simulink library "sm_trackV_lib_belt_underc_elem"  (R2026a)
settings: Solver=VariableStepAuto
undefined symbols (not defined in the file): Excv, P00, P01, P02, P03, P04, P05, P06, P07, P08, P09, P10, P11, P12, P13, P14, P15, P16, P17, P18, P19, P20, Trac, X, Y, Z
libraries: sm_lib x193, $bdroot x42
(part 3 of 5)

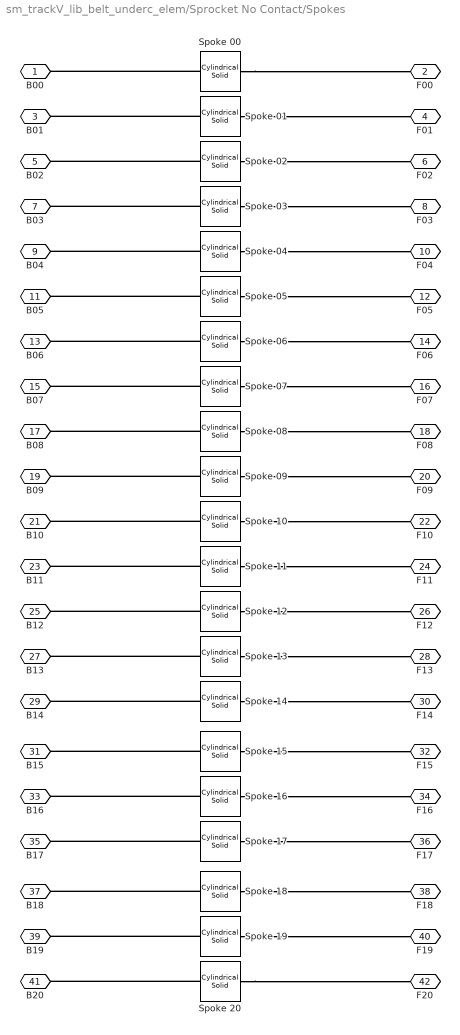
== system sm_trackV_lib_belt_underc_elem/Sprocket No Contact/Spokes ==
  Spoke 00 : sm_lib/Body Elements/Cylindrical Solid  CylinderRadius=sprk_spoke_rad  CylinderRadiusUnits=m  CylinderLength=sprk_spoke_len  CylinderLengthUnits=m  ExportEntireGeometry=off  InertiaType=PointMass  BasedOnType=Density  Density=1000  DensityUnits=kg/m^3  Mass=0  MassUnits=kg  CenterOfMass=[0 0 0]  CenterOfMassUnits=m  MomentsOfInertia=[1 1 1]  MomentsOfInertiaUnits=kg*m^2  ProductsOfInertia=[0 0 0]  ProductsOfInertiaUnits=kg*m^2  GraphicType=FromGeometry  MarkerShape=Sphere  MarkerSize=10  GraphicVisPropType=SimpleVisualProperties  GraphicDiffuseColor=sprk_spoke_clr  GraphicOpacity=sprk_spoke_opc  GraphicSpecularColor=[0.5 0.5 0.5 1.0]  GraphicAmbientColor=[0.15 0.15 0.15 1.0]  GraphicEmissiveColor=[0.0 0.0 0.0 1.0]  GraphicShininess=75  DoExposeReferenceFrame=on  SerializedFrames=<Frames><Frame><Id>Frame1</Id><Value><Name>C</Name><Origin><Source>GeometricFeature</Source><FeatureName>side surface</FeatureName></Origin><PrimaryAxis><DefinedDirection>+Z</DefinedDirection><Source>ReferenceFrame</Source><SourceDirection>+Z</SourceDirection><FeatureName></FeatureName></PrimaryAxis><SecondaryAxis><DefinedDirection>+X</DefinedDirection><Source>ReferenceFrame</Source><SourceDirection>+X</SourceDirection><FeatureName></FeatureName></SecondaryAxis></Value></Frame></Frames>
  Spoke 01 : sm_lib/Body Elements/Cylindrical Solid  CylinderRadius=sprk_spoke_rad  CylinderRadiusUnits=m  CylinderLength=sprk_spoke_len  CylinderLengthUnits=m  ExportEntireGeometry=off  InertiaType=PointMass  BasedOnType=Density  Density=1000  DensityUnits=kg/m^3  Mass=0  MassUnits=kg  CenterOfMass=[0 0 0]  CenterOfMassUnits=m  MomentsOfInertia=[1 1 1]  MomentsOfInertiaUnits=kg*m^2  ProductsOfInertia=[0 0 0]  ProductsOfInertiaUnits=kg*m^2  GraphicType=FromGeometry  MarkerShape=Sphere  MarkerSize=10  GraphicVisPropType=SimpleVisualProperties  GraphicDiffuseColor=sprk_spoke_clr  GraphicOpacity=sprk_spoke_opc  GraphicSpecularColor=[0.5 0.5 0.5 1.0]  GraphicAmbientColor=[0.15 0.15 0.15 1.0]  GraphicEmissiveColor=[0.0 0.0 0.0 1.0]  GraphicShininess=75  DoExposeReferenceFrame=on  SerializedFrames=<Frames><Frame><Id>Frame1</Id><Value><Name>C</Name><Origin><Source>GeometricFeature</Source><FeatureName>side surface</FeatureName></Origin><PrimaryAxis><DefinedDirection>+Z</DefinedDirection><Source>ReferenceFrame</Source><SourceDirection>+Z</SourceDirection><FeatureName></FeatureName></PrimaryAxis><SecondaryAxis><DefinedDirection>+X</DefinedDirection><Source>ReferenceFrame</Source><SourceDirection>+X</SourceDirection><FeatureName></FeatureName></SecondaryAxis></Value></Frame></Frames>
  Spoke 02 : sm_lib/Body Elements/Cylindrical Solid  CylinderRadius=sprk_spoke_rad  CylinderRadiusUnits=m  CylinderLength=sprk_spoke_len  CylinderLengthUnits=m  ExportEntireGeometry=off  InertiaType=PointMass  BasedOnType=Density  Density=1000  DensityUnits=kg/m^3  Mass=0  MassUnits=kg  CenterOfMass=[0 0 0]  CenterOfMassUnits=m  MomentsOfInertia=[1 1 1]  MomentsOfInertiaUnits=kg*m^2  ProductsOfInertia=[0 0 0]  ProductsOfInertiaUnits=kg*m^2  GraphicType=FromGeometry  MarkerShape=Sphere  MarkerSize=10  GraphicVisPropType=SimpleVisualProperties  GraphicDiffuseColor=sprk_spoke_clr  GraphicOpacity=sprk_spoke_opc  GraphicSpecularColor=[0.5 0.5 0.5 1.0]  GraphicAmbientColor=[0.15 0.15 0.15 1.0]  GraphicEmissiveColor=[0.0 0.0 0.0 1.0]  GraphicShininess=75  DoExposeReferenceFrame=on  SerializedFrames=<Frames><Frame><Id>Frame1</Id><Value><Name>C</Name><Origin><Source>GeometricFeature</Source><FeatureName>side surface</FeatureName></Origin><PrimaryAxis><DefinedDirection>+Z</DefinedDirection><Source>ReferenceFrame</Source><SourceDirection>+Z</SourceDirection><FeatureName></FeatureName></PrimaryAxis><SecondaryAxis><DefinedDirection>+X</DefinedDirection><Source>ReferenceFrame</Source><SourceDirection>+X</SourceDirection><FeatureName></FeatureName></SecondaryAxis></Value></Frame></Frames>
  Spoke 03 : sm_lib/Body Elements/Cylindrical Solid  CylinderRadius=sprk_spoke_rad  CylinderRadiusUnits=m  CylinderLength=sprk_spoke_len  CylinderLengthUnits=m  ExportEntireGeometry=off  InertiaType=PointMass  BasedOnType=Density  Density=1000  DensityUnits=kg/m^3  Mass=0  MassUnits=kg  CenterOfMass=[0 0 0]  CenterOfMassUnits=m  MomentsOfInertia=[1 1 1]  MomentsOfInertiaUnits=kg*m^2  ProductsOfInertia=[0 0 0]  ProductsOfInertiaUnits=kg*m^2  GraphicType=FromGeometry  MarkerShape=Sphere  MarkerSize=10  GraphicVisPropType=SimpleVisualProperties  GraphicDiffuseColor=sprk_spoke_clr  GraphicOpacity=sprk_spoke_opc  GraphicSpecularColor=[0.5 0.5 0.5 1.0]  GraphicAmbientColor=[0.15 0.15 0.15 1.0]  GraphicEmissiveColor=[0.0 0.0 0.0 1.0]  GraphicShininess=75  DoExposeReferenceFrame=on  SerializedFrames=<Frames><Frame><Id>Frame1</Id><Value><Name>C</Name><Origin><Source>GeometricFeature</Source><FeatureName>side surface</FeatureName></Origin><PrimaryAxis><DefinedDirection>+Z</DefinedDirection><Source>ReferenceFrame</Source><SourceDirection>+Z</SourceDirection><FeatureName></FeatureName></PrimaryAxis><SecondaryAxis><DefinedDirection>+X</DefinedDirection><Source>ReferenceFrame</Source><SourceDirection>+X</SourceDirection><FeatureName></FeatureName></SecondaryAxis></Value></Frame></Frames>
  Spoke 04 : sm_lib/Body Elements/Cylindrical Solid  CylinderRadius=sprk_spoke_rad  CylinderRadiusUnits=m  CylinderLength=sprk_spoke_len  CylinderLengthUnits=m  ExportEntireGeometry=off  InertiaType=PointMass  BasedOnType=Density  Density=1000  DensityUnits=kg/m^3  Mass=0  MassUnits=kg  CenterOfMass=[0 0 0]  CenterOfMassUnits=m  MomentsOfInertia=[1 1 1]  MomentsOfInertiaUnits=kg*m^2  ProductsOfInertia=[0 0 0]  ProductsOfInertiaUnits=kg*m^2  GraphicType=FromGeometry  MarkerShape=Sphere  MarkerSize=10  GraphicVisPropType=SimpleVisualProperties  GraphicDiffuseColor=sprk_spoke_clr  GraphicOpacity=sprk_spoke_opc  GraphicSpecularColor=[0.5 0.5 0.5 1.0]  GraphicAmbientColor=[0.15 0.15 0.15 1.0]  GraphicEmissiveColor=[0.0 0.0 0.0 1.0]  GraphicShininess=75  DoExposeReferenceFrame=on  SerializedFrames=<Frames><Frame><Id>Frame1</Id><Value><Name>C</Name><Origin><Source>GeometricFeature</Source><FeatureName>side surface</FeatureName></Origin><PrimaryAxis><DefinedDirection>+Z</DefinedDirection><Source>ReferenceFrame</Source><SourceDirection>+Z</SourceDirection><FeatureName></FeatureName></PrimaryAxis><SecondaryAxis><DefinedDirection>+X</DefinedDirection><Source>ReferenceFrame</Source><SourceDirection>+X</SourceDirection><FeatureName></FeatureName></SecondaryAxis></Value></Frame></Frames>
  Spoke 05 : sm_lib/Body Elements/Cylindrical Solid  CylinderRadius=sprk_spoke_rad  CylinderRadiusUnits=m  CylinderLength=sprk_spoke_len  CylinderLengthUnits=m  ExportEntireGeometry=off  InertiaType=PointMass  BasedOnType=Density  Density=1000  DensityUnits=kg/m^3  Mass=0  MassUnits=kg  CenterOfMass=[0 0 0]  CenterOfMassUnits=m  MomentsOfInertia=[1 1 1]  MomentsOfInertiaUnits=kg*m^2  ProductsOfInertia=[0 0 0]  ProductsOfInertiaUnits=kg*m^2  GraphicType=FromGeometry  MarkerShape=Sphere  MarkerSize=10  GraphicVisPropType=SimpleVisualProperties  GraphicDiffuseColor=sprk_spoke_clr  GraphicOpacity=sprk_spoke_opc  GraphicSpecularColor=[0.5 0.5 0.5 1.0]  GraphicAmbientColor=[0.15 0.15 0.15 1.0]  GraphicEmissiveColor=[0.0 0.0 0.0 1.0]  GraphicShininess=75  DoExposeReferenceFrame=on  SerializedFrames=<Frames><Frame><Id>Frame1</Id><Value><Name>C</Name><Origin><Source>GeometricFeature</Source><FeatureName>side surface</FeatureName></Origin><PrimaryAxis><DefinedDirection>+Z</DefinedDirection><Source>ReferenceFrame</Source><SourceDirection>+Z</SourceDirection><FeatureName></FeatureName></PrimaryAxis><SecondaryAxis><DefinedDirection>+X</DefinedDirection><Source>ReferenceFrame</Source><SourceDirection>+X</SourceDirection><FeatureName></FeatureName></SecondaryAxis></Value></Frame></Frames>
  Spoke 06 : sm_lib/Body Elements/Cylindrical Solid  CylinderRadius=sprk_spoke_rad  CylinderRadiusUnits=m  CylinderLength=sprk_spoke_len  CylinderLengthUnits=m  ExportEntireGeometry=off  InertiaType=PointMass  BasedOnType=Density  Density=1000  DensityUnits=kg/m^3  Mass=0  MassUnits=kg  CenterOfMass=[0 0 0]  CenterOfMassUnits=m  MomentsOfInertia=[1 1 1]  MomentsOfInertiaUnits=kg*m^2  ProductsOfInertia=[0 0 0]  ProductsOfInertiaUnits=kg*m^2  GraphicType=FromGeometry  MarkerShape=Sphere  MarkerSize=10  GraphicVisPropType=SimpleVisualProperties  GraphicDiffuseColor=sprk_spoke_clr  GraphicOpacity=sprk_spoke_opc  GraphicSpecularColor=[0.5 0.5 0.5 1.0]  GraphicAmbientColor=[0.15 0.15 0.15 1.0]  GraphicEmissiveColor=[0.0 0.0 0.0 1.0]  GraphicShininess=75  DoExposeReferenceFrame=on  SerializedFrames=<Frames><Frame><Id>Frame1</Id><Value><Name>C</Name><Origin><Source>GeometricFeature</Source><FeatureName>side surface</FeatureName></Origin><PrimaryAxis><DefinedDirection>+Z</DefinedDirection><Source>ReferenceFrame</Source><SourceDirection>+Z</SourceDirection><FeatureName></FeatureName></PrimaryAxis><SecondaryAxis><DefinedDirection>+X</DefinedDirection><Source>ReferenceFrame</Source><SourceDirection>+X</SourceDirection><FeatureName></FeatureName></SecondaryAxis></Value></Frame></Frames>
  Spoke 07 : sm_lib/Body Elements/Cylindrical Solid  CylinderRadius=sprk_spoke_rad  CylinderRadiusUnits=m  CylinderLength=sprk_spoke_len  CylinderLengthUnits=m  ExportEntireGeometry=off  InertiaType=PointMass  BasedOnType=Density  Density=1000  DensityUnits=kg/m^3  Mass=0  MassUnits=kg  CenterOfMass=[0 0 0]  CenterOfMassUnits=m  MomentsOfInertia=[1 1 1]  MomentsOfInertiaUnits=kg*m^2  ProductsOfInertia=[0 0 0]  ProductsOfInertiaUnits=kg*m^2  GraphicType=FromGeometry  MarkerShape=Sphere  MarkerSize=10  GraphicVisPropType=SimpleVisualProperties  GraphicDiffuseColor=sprk_spoke_clr  GraphicOpacity=sprk_spoke_opc  GraphicSpecularColor=[0.5 0.5 0.5 1.0]  GraphicAmbientColor=[0.15 0.15 0.15 1.0]  GraphicEmissiveColor=[0.0 0.0 0.0 1.0]  GraphicShininess=75  DoExposeReferenceFrame=on  SerializedFrames=<Frames><Frame><Id>Frame1</Id><Value><Name>C</Name><Origin><Source>GeometricFeature</Source><FeatureName>side surface</FeatureName></Origin><PrimaryAxis><DefinedDirection>+Z</DefinedDirection><Source>ReferenceFrame</Source><SourceDirection>+Z</SourceDirection><FeatureName></FeatureName></PrimaryAxis><SecondaryAxis><DefinedDirection>+X</DefinedDirection><Source>ReferenceFrame</Source><SourceDirection>+X</SourceDirection><FeatureName></FeatureName></SecondaryAxis></Value></Frame></Frames>
  Spoke 08 : sm_lib/Body Elements/Cylindrical Solid  CylinderRadius=sprk_spoke_rad  CylinderRadiusUnits=m  CylinderLength=sprk_spoke_len  CylinderLengthUnits=m  ExportEntireGeometry=off  InertiaType=PointMass  BasedOnType=Density  Density=1000  DensityUnits=kg/m^3  Mass=0  MassUnits=kg  CenterOfMass=[0 0 0]  CenterOfMassUnits=m  MomentsOfInertia=[1 1 1]  MomentsOfInertiaUnits=kg*m^2  ProductsOfInertia=[0 0 0]  ProductsOfInertiaUnits=kg*m^2  GraphicType=FromGeometry  MarkerShape=Sphere  MarkerSize=10  GraphicVisPropType=SimpleVisualProperties  GraphicDiffuseColor=sprk_spoke_clr  GraphicOpacity=sprk_spoke_opc  GraphicSpecularColor=[0.5 0.5 0.5 1.0]  GraphicAmbientColor=[0.15 0.15 0.15 1.0]  GraphicEmissiveColor=[0.0 0.0 0.0 1.0]  GraphicShininess=75  DoExposeReferenceFrame=on  SerializedFrames=<Frames><Frame><Id>Frame1</Id><Value><Name>C</Name><Origin><Source>GeometricFeature</Source><FeatureName>side surface</FeatureName></Origin><PrimaryAxis><DefinedDirection>+Z</DefinedDirection><Source>ReferenceFrame</Source><SourceDirection>+Z</SourceDirection><FeatureName></FeatureName></PrimaryAxis><SecondaryAxis><DefinedDirection>+X</DefinedDirection><Source>ReferenceFrame</Source><SourceDirection>+X</SourceDirection><FeatureName></FeatureName></SecondaryAxis></Value></Frame></Frames>
  Spoke 09 : sm_lib/Body Elements/Cylindrical Solid  CylinderRadius=sprk_spoke_rad  CylinderRadiusUnits=m  CylinderLength=sprk_spoke_len  CylinderLengthUnits=m  ExportEntireGeometry=off  InertiaType=PointMass  BasedOnType=Density  Density=1000  DensityUnits=kg/m^3  Mass=0  MassUnits=kg  CenterOfMass=[0 0 0]  CenterOfMassUnits=m  MomentsOfInertia=[1 1 1]  MomentsOfInertiaUnits=kg*m^2  ProductsOfInertia=[0 0 0]  ProductsOfInertiaUnits=kg*m^2  GraphicType=FromGeometry  MarkerShape=Sphere  MarkerSize=10  GraphicVisPropType=SimpleVisualProperties  GraphicDiffuseColor=sprk_spoke_clr  GraphicOpacity=sprk_spoke_opc  GraphicSpecularColor=[0.5 0.5 0.5 1.0]  GraphicAmbientColor=[0.15 0.15 0.15 1.0]  GraphicEmissiveColor=[0.0 0.0 0.0 1.0]  GraphicShininess=75  DoExposeReferenceFrame=on  SerializedFrames=<Frames><Frame><Id>Frame1</Id><Value><Name>C</Name><Origin><Source>GeometricFeature</Source><FeatureName>side surface</FeatureName></Origin><PrimaryAxis><DefinedDirection>+Z</DefinedDirection><Source>ReferenceFrame</Source><SourceDirection>+Z</SourceDirection><FeatureName></FeatureName></PrimaryAxis><SecondaryAxis><DefinedDirection>+X</DefinedDirection><Source>ReferenceFrame</Source><SourceDirection>+X</SourceDirection><FeatureName></FeatureName></SecondaryAxis></Value></Frame></Frames>
  Spoke {10..20} (11 alike) : sm_lib/Body Elements/Cylindrical Solid  CylinderRadius=sprk_spoke_rad  CylinderRadiusUnits=m  CylinderLength=sprk_spoke_len  CylinderLengthUnits=m  ExportEntireGeometry=off  InertiaType=PointMass  BasedOnType=Density  Density=1000  DensityUnits=kg/m^3  Mass=0  MassUnits=kg  CenterOfMass=[0 0 0]  CenterOfMassUnits=m  MomentsOfInertia=[1 1 1]  MomentsOfInertiaUnits=kg*m^2  ProductsOfInertia=[0 0 0]  ProductsOfInertiaUnits=kg*m^2  GraphicType=FromGeometry  MarkerShape=Sphere  MarkerSize=10  GraphicVisPropType=SimpleVisualProperties  GraphicDiffuseColor=sprk_spoke_clr  GraphicOpacity=sprk_spoke_opc  GraphicSpecularColor=[0.5 0.5 0.5 1.0]  GraphicAmbientColor=[0.15 0.15 0.15 1.0]  GraphicEmissiveColor=[0.0 0.0 0.0 1.0]  GraphicShininess=75  DoExposeReferenceFrame=on  SerializedFrames=<Frames><Frame><Id>Frame1</Id><Value><Name>C</Name><Origin><Source>GeometricFeature</Source><FeatureName>side surface</FeatureName></Origin><PrimaryAxis><DefinedDirection>+Z</DefinedDirection><Source>ReferenceFrame</Source><SourceDirection>+Z</SourceDirection><FeatureName></FeatureName></PrimaryAxis><SecondaryAxis><DefinedDirection>+X</DefinedDirection><Source>ReferenceFrame</Source><SourceDirection>+X</SourceDirection><FeatureName></FeatureName></SecondaryAxis></Value></Frame></Frames>
  B00 : PMIOPort  Side=Left
  F00 : PMIOPort  Port=2  Side=Right
  B01 : PMIOPort  Port=3  Side=Left
  F01 : PMIOPort  Port=4  Side=Right
  B02 : PMIOPort  Port=5  Side=Left
  F02 : PMIOPort  Port=6  Side=Right
  B03 : PMIOPort  Port=7  Side=Left
  F03 : PMIOPort  Port=8  Side=Right
  B04 : PMIOPort  Port=9  Side=Left
  F04 : PMIOPort  Port=10  Side=Right
  B05 : PMIOPort  Port=11  Side=Left
  F05 : PMIOPort  Port=12  Side=Right
  B06 : PMIOPort  Port=13  Side=Left
  F06 : PMIOPort  Port=14  Side=Right
  B07 : PMIOPort  Port=15  Side=Left
  F07 : PMIOPort  Port=16  Side=Right
  B08 : PMIOPort  Port=17  Side=Left
  F08 : PMIOPort  Port=18  Side=Right
  B09 : PMIOPort  Port=19  Side=Left
  F09 : PMIOPort  Port=20  Side=Right
  B10 : PMIOPort  Port=21  Side=Left
  F10 : PMIOPort  Port=22  Side=Right
  B11 : PMIOPort  Port=23  Side=Left
  F11 : PMIOPort  Port=24  Side=Right
  B12 : PMIOPort  Port=25  Side=Left
  F12 : PMIOPort  Port=26  Side=Right
  B13 : PMIOPort  Port=27  Side=Left
  F13 : PMIOPort  Port=28  Side=Right
  B14 : PMIOPort  Port=29  Side=Left
  F14 : PMIOPort  Port=30  Side=Right
  B15 : PMIOPort  Port=31  Side=Left
  F15 : PMIOPort  Port=32  Side=Right
  B16 : PMIOPort  Port=33  Side=Left
  F16 : PMIOPort  Port=34  Side=Right
  B17 : PMIOPort  Port=35  Side=Left
  F17 : PMIOPort  Port=36  Side=Right
  B18 : PMIOPort  Port=37  Side=Left
  F18 : PMIOPort  Port=38  Side=Right
  B19 : PMIOPort  Port=39  Side=Left
  F19 : PMIOPort  Port=40  Side=Right
  B20 : PMIOPort  Port=41  Side=Left
  F20 : PMIOPort  Port=42  Side=Right
  connections:
  Spoke 20/RConn1 -- F20/RConn1
  Spoke 08/RConn1 -- F08/RConn1
  Spoke 06/RConn1 -- F06/RConn1
  Spoke 02/RConn1 -- F02/RConn1
  Spoke 04/RConn1 -- F04/RConn1
  Spoke 14/RConn1 -- F14/RConn1
  Spoke 03/RConn1 -- F03/RConn1
  Spoke 17/RConn1 -- F17/RConn1
  Spoke 15/LConn1 -- B15/RConn1
  Spoke 20/LConn1 -- B20/RConn1
  Spoke 16/LConn1 -- B16/RConn1
  Spoke 04/LConn1 -- B04/RConn1
  Spoke 05/LConn1 -- B05/RConn1
  Spoke 14/LConn1 -- B14/RConn1
  Spoke 11/RConn1 -- F11/RConn1
  Spoke 11/LConn1 -- B11/RConn1
  Spoke 12/RConn1 -- F12/RConn1
  Spoke 18/RConn1 -- F18/RConn1
  Spoke 13/LConn1 -- B13/RConn1
  Spoke 02/LConn1 -- B02/RConn1
  Spoke 09/LConn1 -- B09/RConn1
  Spoke 19/LConn1 -- B19/RConn1
  Spoke 17/LConn1 -- B17/RConn1
  Spoke 18/LConn1 -- B18/RConn1
  Spoke 19/RConn1 -- F19/RConn1
  Spoke 05/RConn1 -- F05/RConn1
  Spoke 16/RConn1 -- F16/RConn1
  Spoke 09/RConn1 -- F09/RConn1
  Spoke 10/LConn1 -- B10/RConn1
  Spoke 07/LConn1 -- B07/RConn1
  Spoke 10/RConn1 -- F10/RConn1
  Spoke 07/RConn1 -- F07/RConn1
  Spoke 00/RConn1 -- F00/RConn1
  Spoke 01/LConn1 -- B01/RConn1
  Spoke 08/LConn1 -- B08/RConn1
  Spoke 12/LConn1 -- B12/RConn1
  Spoke 01/RConn1 -- F01/RConn1
  Spoke 15/RConn1 -- F15/RConn1
  Spoke 13/RConn1 -- F13/RConn1
  Spoke 06/LConn1 -- B06/RConn1
  Spoke 03/LConn1 -- B03/RConn1
  Spoke 00/LConn1 -- B00/RConn1

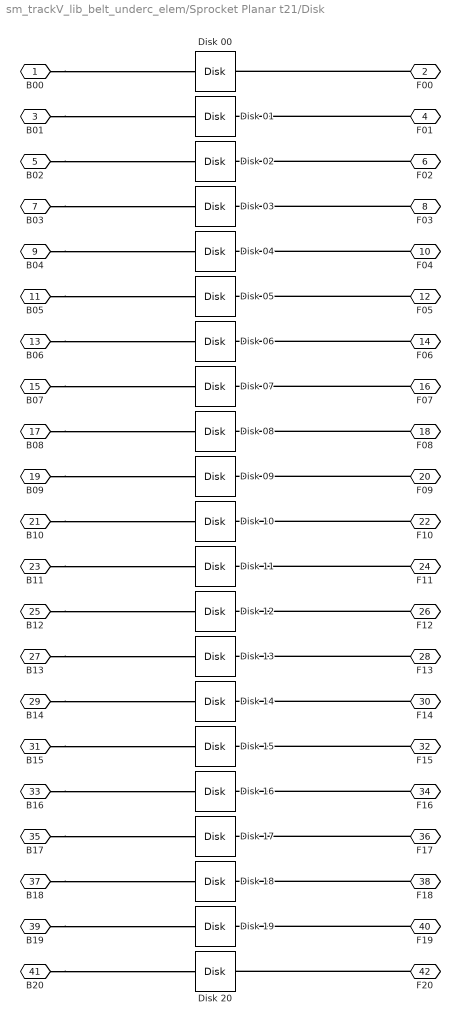
== system sm_trackV_lib_belt_underc_elem/Sprocket Planar t21/Disk ==
  Disk 00 : sm_lib/Curves and Surfaces/Disk  Radius=sprk_spoke_rad  RadiusUnits=m  GraphicType=FromGeometry  GraphicVisPropType=SimpleVisualProperties  GraphicDiffuseColor=sprk_contgeo_spoke_clr  GraphicOpacity=sprk_contgeo_spoke_opc  GraphicSpecularColor=[0.5 0.5 0.5 1.0]  GraphicAmbientColor=[0.15 0.15 0.15 1.0]  GraphicEmissiveColor=[0.0 0.0 0.0 1.0]  GraphicShininess=75
  Disk 01 : sm_lib/Curves and Surfaces/Disk  Radius=sprk_spoke_rad  RadiusUnits=m  GraphicType=FromGeometry  GraphicVisPropType=SimpleVisualProperties  GraphicDiffuseColor=sprk_contgeo_spoke_clr  GraphicOpacity=sprk_contgeo_spoke_opc  GraphicSpecularColor=[0.5 0.5 0.5 1.0]  GraphicAmbientColor=[0.15 0.15 0.15 1.0]  GraphicEmissiveColor=[0.0 0.0 0.0 1.0]  GraphicShininess=75
  Disk 02 : sm_lib/Curves and Surfaces/Disk  Radius=sprk_spoke_rad  RadiusUnits=m  GraphicType=FromGeometry  GraphicVisPropType=SimpleVisualProperties  GraphicDiffuseColor=sprk_contgeo_spoke_clr  GraphicOpacity=sprk_contgeo_spoke_opc  GraphicSpecularColor=[0.5 0.5 0.5 1.0]  GraphicAmbientColor=[0.15 0.15 0.15 1.0]  GraphicEmissiveColor=[0.0 0.0 0.0 1.0]  GraphicShininess=75
  Disk 03 : sm_lib/Curves and Surfaces/Disk  Radius=sprk_spoke_rad  RadiusUnits=m  GraphicType=FromGeometry  GraphicVisPropType=SimpleVisualProperties  GraphicDiffuseColor=sprk_contgeo_spoke_clr  GraphicOpacity=sprk_contgeo_spoke_opc  GraphicSpecularColor=[0.5 0.5 0.5 1.0]  GraphicAmbientColor=[0.15 0.15 0.15 1.0]  GraphicEmissiveColor=[0.0 0.0 0.0 1.0]  GraphicShininess=75
  Disk 04 : sm_lib/Curves and Surfaces/Disk  Radius=sprk_spoke_rad  RadiusUnits=m  GraphicType=FromGeometry  GraphicVisPropType=SimpleVisualProperties  GraphicDiffuseColor=sprk_contgeo_spoke_clr  GraphicOpacity=sprk_contgeo_spoke_opc  GraphicSpecularColor=[0.5 0.5 0.5 1.0]  GraphicAmbientColor=[0.15 0.15 0.15 1.0]  GraphicEmissiveColor=[0.0 0.0 0.0 1.0]  GraphicShininess=75
  Disk 05 : sm_lib/Curves and Surfaces/Disk  Radius=sprk_spoke_rad  RadiusUnits=m  GraphicType=FromGeometry  GraphicVisPropType=SimpleVisualProperties  GraphicDiffuseColor=sprk_contgeo_spoke_clr  GraphicOpacity=sprk_contgeo_spoke_opc  GraphicSpecularColor=[0.5 0.5 0.5 1.0]  GraphicAmbientColor=[0.15 0.15 0.15 1.0]  GraphicEmissiveColor=[0.0 0.0 0.0 1.0]  GraphicShininess=75
  Disk 06 : sm_lib/Curves and Surfaces/Disk  Radius=sprk_spoke_rad  RadiusUnits=m  GraphicType=FromGeometry  GraphicVisPropType=SimpleVisualProperties  GraphicDiffuseColor=sprk_contgeo_spoke_clr  GraphicOpacity=sprk_contgeo_spoke_opc  GraphicSpecularColor=[0.5 0.5 0.5 1.0]  GraphicAmbientColor=[0.15 0.15 0.15 1.0]  GraphicEmissiveColor=[0.0 0.0 0.0 1.0]  GraphicShininess=75
  Disk 07 : sm_lib/Curves and Surfaces/Disk  Radius=sprk_spoke_rad  RadiusUnits=m  GraphicType=FromGeometry  GraphicVisPropType=SimpleVisualProperties  GraphicDiffuseColor=sprk_contgeo_spoke_clr  GraphicOpacity=sprk_contgeo_spoke_opc  GraphicSpecularColor=[0.5 0.5 0.5 1.0]  GraphicAmbientColor=[0.15 0.15 0.15 1.0]  GraphicEmissiveColor=[0.0 0.0 0.0 1.0]  GraphicShininess=75
  Disk 08 : sm_lib/Curves and Surfaces/Disk  Radius=sprk_spoke_rad  RadiusUnits=m  GraphicType=FromGeometry  GraphicVisPropType=SimpleVisualProperties  GraphicDiffuseColor=sprk_contgeo_spoke_clr  GraphicOpacity=sprk_contgeo_spoke_opc  GraphicSpecularColor=[0.5 0.5 0.5 1.0]  GraphicAmbientColor=[0.15 0.15 0.15 1.0]  GraphicEmissiveColor=[0.0 0.0 0.0 1.0]  GraphicShininess=75
  Disk 09 : sm_lib/Curves and Surfaces/Disk  Radius=sprk_spoke_rad  RadiusUnits=m  GraphicType=FromGeometry  GraphicVisPropType=SimpleVisualProperties  GraphicDiffuseColor=sprk_contgeo_spoke_clr  GraphicOpacity=sprk_contgeo_spoke_opc  GraphicSpecularColor=[0.5 0.5 0.5 1.0]  GraphicAmbientColor=[0.15 0.15 0.15 1.0]  GraphicEmissiveColor=[0.0 0.0 0.0 1.0]  GraphicShininess=75
  Disk {10..20} (11 alike) : sm_lib/Curves and Surfaces/Disk  Radius=sprk_spoke_rad  RadiusUnits=m  GraphicType=FromGeometry  GraphicVisPropType=SimpleVisualProperties  GraphicDiffuseColor=sprk_contgeo_spoke_clr  GraphicOpacity=sprk_contgeo_spoke_opc  GraphicSpecularColor=[0.5 0.5 0.5 1.0]  GraphicAmbientColor=[0.15 0.15 0.15 1.0]  GraphicEmissiveColor=[0.0 0.0 0.0 1.0]  GraphicShininess=75
  B00 : PMIOPort  Side=Left
  F00 : PMIOPort  Port=2  Side=Right
  B01 : PMIOPort  Port=3  Side=Left
  F01 : PMIOPort  Port=4  Side=Right
  B02 : PMIOPort  Port=5  Side=Left
  F02 : PMIOPort  Port=6  Side=Right
  B03 : PMIOPort  Port=7  Side=Left
  F03 : PMIOPort  Port=8  Side=Right
  B04 : PMIOPort  Port=9  Side=Left
  F04 : PMIOPort  Port=10  Side=Right
  B05 : PMIOPort  Port=11  Side=Left
  F05 : PMIOPort  Port=12  Side=Right
  B06 : PMIOPort  Port=13  Side=Left
  F06 : PMIOPort  Port=14  Side=Right
  B07 : PMIOPort  Port=15  Side=Left
  F07 : PMIOPort  Port=16  Side=Right
  B08 : PMIOPort  Port=17  Side=Left
  F08 : PMIOPort  Port=18  Side=Right
  B09 : PMIOPort  Port=19  Side=Left
  F09 : PMIOPort  Port=20  Side=Right
  B10 : PMIOPort  Port=21  Side=Left
  F10 : PMIOPort  Port=22  Side=Right
  B11 : PMIOPort  Port=23  Side=Left
  F11 : PMIOPort  Port=24  Side=Right
  B12 : PMIOPort  Port=25  Side=Left
  F12 : PMIOPort  Port=26  Side=Right
  B13 : PMIOPort  Port=27  Side=Left
  F13 : PMIOPort  Port=28  Side=Right
  B14 : PMIOPort  Port=29  Side=Left
  F14 : PMIOPort  Port=30  Side=Right
  B15 : PMIOPort  Port=31  Side=Left
  F15 : PMIOPort  Port=32  Side=Right
  B16 : PMIOPort  Port=33  Side=Left
  F16 : PMIOPort  Port=34  Side=Right
  B17 : PMIOPort  Port=35  Side=Left
  F17 : PMIOPort  Port=36  Side=Right
  B18 : PMIOPort  Port=37  Side=Left
  F18 : PMIOPort  Port=38  Side=Right
  B19 : PMIOPort  Port=39  Side=Left
  F19 : PMIOPort  Port=40  Side=Right
  B20 : PMIOPort  Port=41  Side=Left
  F20 : PMIOPort  Port=42  Side=Right
  connections:
  B01/RConn1 -- Disk 01/LConn1
  F10/RConn1 -- Disk 10/RConn1
  B13/RConn1 -- Disk 13/LConn1
  B05/RConn1 -- Disk 05/LConn1
  B06/RConn1 -- Disk 06/LConn1
  B00/RConn1 -- Disk 00/LConn1
  F00/RConn1 -- Disk 00/RConn1
  B19/RConn1 -- Disk 19/LConn1
  B14/RConn1 -- Disk 14/LConn1
  B20/RConn1 -- Disk 20/LConn1
  B02/RConn1 -- Disk 02/LConn1
  B04/RConn1 -- Disk 04/LConn1
  B03/RConn1 -- Disk 03/LConn1
  B07/RConn1 -- Disk 07/LConn1
  F11/RConn1 -- Disk 11/RConn1
  B08/RConn1 -- Disk 08/LConn1
  F08/RConn1 -- Disk 08/RConn1
  B12/RConn1 -- Disk 12/LConn1
  B10/RConn1 -- Disk 10/LConn1
  B17/RConn1 -- Disk 17/LConn1
  B09/RConn1 -- Disk 09/LConn1
  B11/RConn1 -- Disk 11/LConn1
  B15/RConn1 -- Disk 15/LConn1
  F04/RConn1 -- Disk 04/RConn1
  B16/RConn1 -- Disk 16/LConn1
  F02/RConn1 -- Disk 02/RConn1
  F07/RConn1 -- Disk 07/RConn1
  F18/RConn1 -- Disk 18/RConn1
  B18/RConn1 -- Disk 18/LConn1
  F17/RConn1 -- Disk 17/RConn1
  F15/RConn1 -- Disk 15/RConn1
  F01/RConn1 -- Disk 01/RConn1
  F16/RConn1 -- Disk 16/RConn1
  F06/RConn1 -- Disk 06/RConn1
  F03/RConn1 -- Disk 03/RConn1
  F20/RConn1 -- Disk 20/RConn1
  F14/RConn1 -- Disk 14/RConn1
  F19/RConn1 -- Disk 19/RConn1
  F09/RConn1 -- Disk 09/RConn1
  F13/RConn1 -- Disk 13/RConn1
  F05/RConn1 -- Disk 05/RConn1
  F12/RConn1 -- Disk 12/RConn1
